simulink model "stm32f4_customcode_demo"  (Simulink 7.3)
settings: Solver=FixedStepDiscrete  SolverMode=SingleTasking  StartTime=0.0  StopTime=10.0  RelTol=1e-3
PreLoadFcn:
  | waijung.modelPreload; % Required for working with Waijung Blockset. Do not remove.
undefined symbols (not defined in the file): HSEOSC, Link, LQFP176, ST, STM32F417IG
libraries: stm32f4_io_lib x2, stm32f4_device_config_lib x1
CloseFcn:
  | waijung.modelClose; % Required for working with Waijung Blockset. Do not remove.
settings Model: Creator=Krisada  LastModifiedBy=Krisada
settings OptimizationCC: OptimizeModelRefInitCode=on  LifeSpan=1
settings HardwareCC: ProdEndianess=LittleEndian  ProdHWDeviceType=ARM Compatible->Cortex - M4  TargetEndianess=LittleEndian  TargetHWDeviceType=ARM Compatible->Cortex - M4
settings RTWCC: SystemTargetFile=stm32f4.tlc  GenerateMakefile=off  TemplateMakefile=ert_default_tmf  Description=STM32F4 Target  RetainRTWFile=on  ProcessScript=stm32f4_make_rtw_hook
settings CodeAppCC: IgnoreCustomStorageClasses=off
settings STFCustomTargetCC: ModelReferenceCompliant=off  CombineOutputUpdateFcns=on  ERTCustomFileBanners=on  SupportContinuousTime=off  SupportNonInlinedSFcns=off  SystemTargetFile=stm32f4.tlc
settings ERTTargetCC: MultiwordLength=2048  ModelReferenceCompliant=off  ParMdlRefBuildCompliant=off  CompOptLevelCompliant=off  ERTFirstTimeCompliant=off  ModelStepFunctionPrototypeControlCompliant=off  CPPClassGenCompliant=off  InlinedParameterPlacement=NonHierarchical  ERTSrcFileBannerTemplate=stm32f4_code_template.cgt  ERTHdrFileBannerTemplate=stm32f4_code_template.cgt  ERTDataSrcFileTemplate=stm32f4_code_template.cgt  ERTDataHdrFileTemplate=stm32f4_code_template.cgt  ERTCustomFileTemplate=stm32f4_file_process.tlc

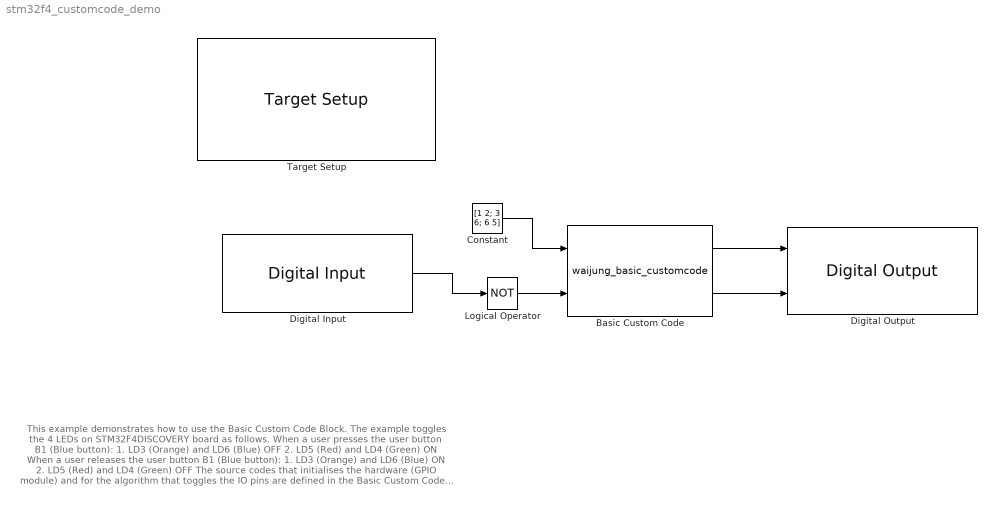
== system stm32f4_customcode_demo ==
  note: This example demonstrates how to use the Basic Custom Code Block. The example toggles the 4 LEDs on STM32F4DISCOVERY board as follows.
      | When a user presses the user button B1 (Blue button):
      | 1. LD3 (Orange) and LD6 (Blue) OFF
      | 2. LD5 (Red) and LD4 (Green) ON
      | When a user releases the user button B1 (Blue button):
      | 1. LD3 (Orange) and LD6 (Blue) ON
      | 2. LD5 (Red) and LD4 (Green) OFF
      |
      | The source codes that initialises the hardware (GPIO module) and for the algorithm that toggles the IO pins are defined in the Basic Custom Code Block.
      | Note: PA0 of STM32F4DISCOVERY is connected to the user button.
  Basic Custom Code : S-Function  FunctionName=waijung_basic_customcode  Parameters=inputportcount,inputporttypeid,outputportcount,outputporttypeid,sampletime,blockid,cinputportlabelstr,coutputportlabelstr,incfilestrarray,outputporttype,inputporttype,initialfuncallstr,enablefuncallstr,outputfuncallstr,disablefuncallstr,inputportdiminfo,outputportdiminfo  EnableBusSupport=off  mask(waijung_basic_customcode){inputporttype=double,boolean, cinputportlabel=to PD12, to PD13, cinputportlabelstr=["to PD12"," to PD13"], inputportcount=2, inputporttypeid=[0  8], outputporttype=boolean,boolean, coutputportlabel=NonInvOut, InvOut, coutputportlabelstr=["NonInvOut"," InvOut"], outputportcount=2, outputporttypeid=[8  8], incpath={fullfile(pwd,'customcode')}, srcpath={fullfile(pwd,'customcode')}, incfiles={'stm32f4_io_customcode.h'}, srcfiles={'stm32f4_io_customcode.c'}, initialfuncallstr=start_customio();, enablefuncallstr=enable_customio();, outputfuncallstr=output_customio(in1,in2,out1,out2);, disablefuncallstr=disable_customio();, sampletime=-1, sampletimestr=0.01, blockid=BasicCustomCode, enablecustomportlabel=on, incfilestrarray=["stm32f4_io_customcode.h"], inputportdiminfo=[1  1  1  0;1  1  1  8], outputportdiminfo=[1  1  1  8;1  1  1  8]}
      mask prompts: inputporttype "Input port definition (data type) separted by comma e.g. double, single, double, uint8"; cinputportlabel "Custom input port labels (Ex. In1, In2, In3)"; cinputportlabelstr "Custom input port type string"; inputportcount "Input port count"; inputporttypeid "Input port data type ID"; outputporttype "Output port definition  (data type) separted by comma e.g. double, single, double, uint8"; coutputportlabel "Custom output port labels (Ex. Out1, Out2, Out3)"; coutputportlabelstr "Custom output port type string"; outputportcount "Output port count"; outputporttypeid "Output port data type ID"; incpath "Path for include files (*.h), defined as cell array of string."; srcpath "Path for source files (*.c), defined as cell array of string."; incfiles "Included header file names with extension (.h), defined as cell array of string."; srcfiles "Included source file names with extension (.c), defined as cell array of string."; initialfuncallstr "Initial function call string"; enablefuncallstr "Enable function call string"; outputfuncallstr "Output function call string"; disablefuncallstr "Disable function call string"; sampletime "Sample time (sec)"; sampletimestr "Sample time string"; blockid "Block ID"; enablecustomportlabel "Enable custom port labels"; incfilestrarray "Header file array"; inputportdiminfo "Input Port Dimension Information (Define in cmex)"; outputportdiminfo "Output Port Dimension Information"
      mask help:
      | This block implements a basic custom code block.
      |
      | Allowed input/output datatype:
      | dynamic,double,single,int8,uint8,int16,uint16,int32,uint32,boolean. Leave this field empty if no input or output needed.
      |
      | "Path for include files" defines the include path. All *.h files in these path(s) will be used in the build process.
      |
      | "Path for source files" defines path to look for each source file(s) defined in the "Included source file name ...". All required source file(s) and source file path(s) must be explicitly defined.
      |
      | "Included header file names ..." field is used to list any *.h file that will be included in #include statements of waijung_hwdrvlib.h.
      |
      | The Basic Custom Code Block supports 2-D input/output matrix/vector signals.
      |
      | The dimensions of input signals are automatically inherited from the supplied input signals.
      | The dimensions of output signals must be implicitly defined using the following format.
      |
      | DataType:nRowsxnCols
      |
      | If dimensions are not defined, scalar signal (1x1) is assumed.
      |
      | For examples: double:4x5,int8,int16:3x1
      mask init:
      | waijung_basic_customcode_callback('init');
      mask Help: web(fullfile(waijungdocroot,'waijung_basic_customcode.htm'), '-browser')
      mask CallbackString: waijung_basic_customcode_callback('inputporttype');|waijung_basic_customcode_callback('cinputportlabel');||||waijung_basic_customcode_callback('outputporttype');|waijung_basic_customcode_callback('coutputportlabel');||||||waijung_basic_customcode_callback('incfiles');||||||waijung_basic_customcode_callback('sampletime');||waijung_basic_customcode_callback('blockid');||||
      mask Display: text(0.5, 0.5, 'Ts (sec): 0.01','ver','middle','hor','center');port_label('input', 1,'to PD12');port_label('input', 2,'to PD13');port_label('output', 1,'NonInvOut');port_label('output', 2,'InvOut')
  Constant : Constant  Value=[1 2; 3 6; 6 5]  OutDataType=fixdt(1, 16)  OutScaling=2^0
  Digital Input : stm32f4_io_lib/Digital Input  port=A  speed=100  porttype=None  porttypestr=NOPULL  use_pin0=on  use_pin1=off  use_pin2=off  use_pin3=off  use_pin4=off  use_pin5=off  use_pin6=off  use_pin7=off  use_pin8=off  use_pin9=off  use_pin10=off  use_pin11=off  use_pin12=off  use_pin13=off  use_pin14=off  use_pin15=off  pinstr=GPIO_Pin_0  usedpinarray="[1  0  0  0  0  0  0  0  0  0  0  0  0  0  0  0]"  bitbandingstr="#define DigitalInput_A0 Peripheral_BB(GPIOA->IDR, 0)  /* Output pin */"  sampletime=0.01  sampletimestr=0.01  blockid=DigitalInput  enablecustomportlabel=off  glabalinit=off  cinputportlabel=In1, In2  coutputportlabel=Out1, Out2
  Digital Output : stm32f4_io_lib/Digital Output  use_bitband=on  port=D  speed=100  porttype=Push Pull  porttypestr=PP  use_pin0=off  use_pin1=off  use_pin2=off  use_pin3=off  use_pin4=off  use_pin5=off  use_pin6=off  use_pin7=off  use_pin8=off  use_pin9=off  use_pin10=off  use_pin11=off  use_pin12=off  use_pin13=off  use_pin14=on  use_pin15=on  pinstr=GPIO_Pin_14 | GPIO_Pin_15  usedpinarray="[0  0  0  0  0  0  0  0  0  0  0  0  0  0  1  1]"  bitbandingstr=|  sampletime=-1  sampletimestr=0.01  blockid=DigitalOutput  enablecustomportlabel=off  globalinit=off  cinputportlabel=In1, In2  coutputportlabel=0
      | #define DigitalOutput_D14 Peripheral_BB(GPIOD->ODR, 14)  /* Output pin */
      | #define DigitalOutput_D15 Peripheral_BB(GPIOD->ODR, 15)  /* Output pin */
  Logical Operator : Logic  Operator=NOT  AllPortsSameDT=off  OutDataTypeMode=boolean  LogicDataType=fixdt(0, 8)  OutDataTypeStr=boolean
  Target Setup : stm32f4_device_config_lib/Target Setup  Priority=100  compiler=GNU ARM  previous_compiler=GNU ARM  mcu=STM32F417IG (LQFP176)  mcustr=STM32F417IG  clockconfig=HSEOSC-8MHz  system_stm32f4xx_c_path=F:\trunk\targets\stm32f4_target\stm32f4\utils\system_stm32f4xx_default\STM32F40_41xxx\hseosc8mhz  showmemoryconfiguration=off  stacksize=0x400  heapsize=0x200  enableautocompiledownload=on  fullchiperase=off  programmerinterface=ST-Link  editctrlstr=on  compilercontrolstr=$(patsubst %, -I%, .) -mcpu=cortex-m4 -mthumb -mthumb-interwork -mfloat-abi=hard -mfpu=fpv4-sp-d16 -ffast-math -Wall -Wextra -Ofast  assemblercontrolstr=$(patsubst %, -I%, .) -mcpu=cortex-m4 -mthumb -mthumb-interwork -mfloat-abi=hard -mfpu=fpv4-sp-d16 -ffast-math -Wall -Wextra -Ofast -Wa,-amhls=$(<:.s=.lst) -D__STACK_SIZE=$(STACK_SIZE) -D__HEAP_SIZE=$(HEAP_SIZE)  linkercontrolstr=-T$(LD_SCRIPT) -g -Wl,-Map=$(MAP),--cref,--no-warn-mismatch -mcpu=cortex-m4 -mthumb -mthumb-interwork -mfloat-abi=hard -mfpu=fpv4-sp-d16 -specs=nosys.specs  runafterdownload=on  execprofile=None  profileruart=1  profilerbaud=115200  profilertxpin=D8  profilerinitstr=0.01,168000000,1680000,115200,0  manualsetsampletime=off  sampletime=0.01  blockid=TargetSetup  systickreloadvalue=1680000  hseval=8000000  lastprofileruart=1  hclk=168000000  flashorigin=0x08000000  flashlength=0x100000  ramorigin=0x20000000  ramlength=0x20000  useextram=off
  wires:
  Digital Input/1 -> Logical Operator/1
  Logical Operator/1 -> Basic Custom Code/2
  Basic Custom Code/1 -> Digital Output/1
  Basic Custom Code/2 -> Digital Output/2
  Constant/1 -> Basic Custom Code/1
